simulink model "Subsystem"  (R2020b)
settings: Solver=FixedStepDiscrete  StartTime=0.0  StopTime=10.0  FixedStep=0.01  RelTol=1e-3
PostLoadFcn:
  | a1=2;
  | a2=-1;
  | b1=1;
  | b2=-1;
model workspace (MAT data in the model file):
  a1 = Simulink.Parameter
  a1.Value = 2
  a1.DataType = 'auto'
  a1.Dimensions = [1 1]
  a2 = Simulink.Parameter
  a2.Value = -1
  a2.DataType = 'auto'
  a2.Dimensions = [1 1]
  b1 = Simulink.Parameter
  b1.Value = 1
  b1.DataType = 'auto'
  b1.Dimensions = [1 1]
  b2 = Simulink.Parameter
  b2.Value = -1
  b2.DataType = 'auto'
  b2.Dimensions = [1 1]
settings Model: Creator=priyaD  LastModifiedBy=priyaD
settings DataIOCC: SaveOutput=off  SaveTime=off

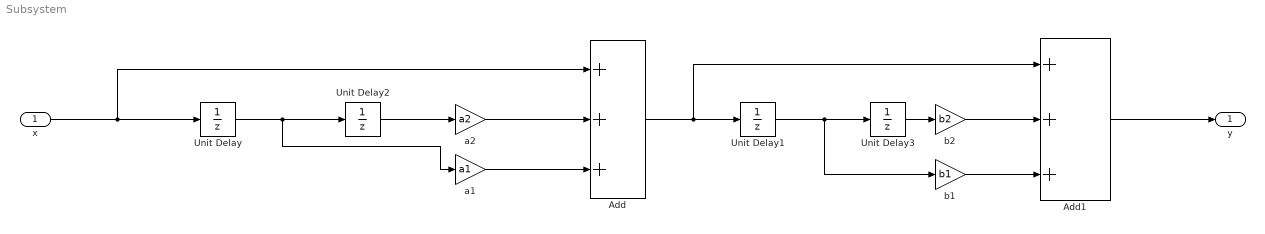
== system Subsystem ==
  x : Inport  OutDataTypeStr=double  PortDimensions=1  SampleTime=0
  Add : Sum  Inputs=+++
  Add1 : Sum  Inputs=+++
  Unit Delay{,1..3} (4 alike) : UnitDelay  SampleTime=-1  HasFrameUpgradeWarning=on
  a1 : Gain  Gain=a1
  a2 : Gain  Gain=a2
  b1 : Gain  Gain=b1
  b2 : Gain  Gain=b2
  y : Outport  OutDataTypeStr=double  PortDimensions=1  SampleTime=0
  wires:
  Add/1 -> Unit Delay1/1, Add1/1
  Unit Delay2/1 -> a2/1
  x/1 -> Unit Delay/1, Add/1
  b1/1 -> Add1/3
  a2/1 -> Add/2
  Unit Delay3/1 -> b2/1
  Add1/1 -> y/1
  b2/1 -> Add1/2
  Unit Delay/1 -> Unit Delay2/1, a1/1
  a1/1 -> Add/3
  Unit Delay1/1 -> Unit Delay3/1, b1/1
